simulink model "wrench_maats_simulator"  (R2025b)
settings: Solver=ode15s  StartTime=0.0  StopTime=100  FixedStep=1e-4  RelTol=1e-3
values from neighbouring files (symbols this model uses):
  Kd1 = 2    [parametrosCarga4x.m]
  x1_0 = xL0+q1_rot*[0;0;L1]    [parametrosCarga4x.m]
  x2_0 = xL0+q2_rot*[0;0;L2]    [parametrosCarga4x.m]
  x3_0 = xL0+q3_rot*[0;0;L3]    [parametrosCarga4x.m]
  x4_0 = xL0+q4_rot*[0;0;L4]    [parametrosCarga4x.m]
  xL0 = [0.8;0.8;0.1]    [parametrosCarga4x.m]
settings Model: Creator=ateveraz  LastModifiedBy=ateveraz

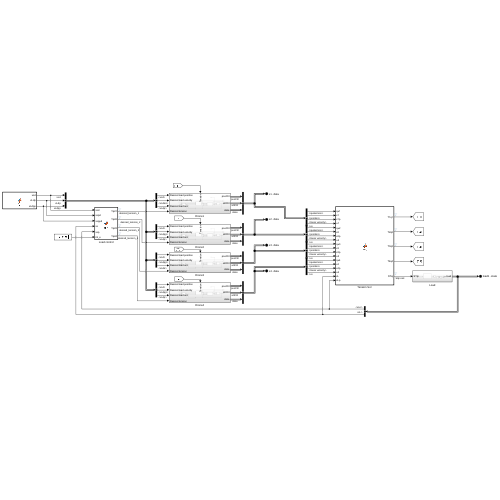
[thumbnail: Simulink's stored preview of the top-level diagram]
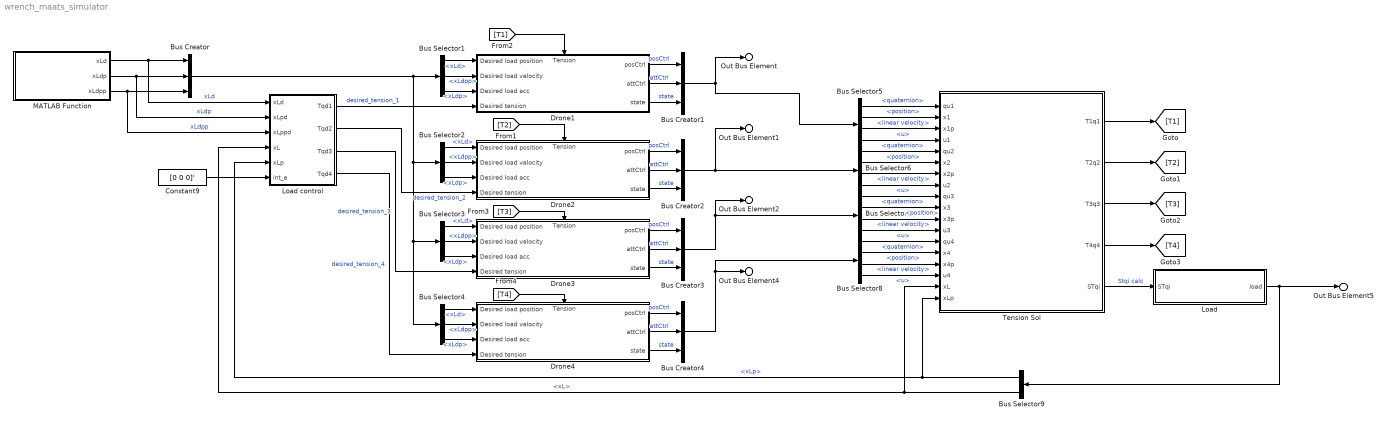
== system wrench_maats_simulator ==
  Bus Creator{,1..4} (5 alike) : BusCreator  Inputs=3
  Bus Selector{1..4} (4 alike) : BusSelector  OutputSignals=xLd,xLdpp,xLdp
  Bus Selector{5..8} (4 alike) : BusSelector  OutputSignals=state.quaternion,state.position,state.linear velocity,posCtrl.u
  Bus Selector9 : BusSelector  OutputSignals=xLp,xL
  Constant9 : Constant  Value=[0 0 0]'
  Drone1 : Subsystem
      settings: PortSchema="{\"entries\":[{\"content\":{\"sides\":[{\"content\":{\"connectorIds\":[\"In1\",\"In2\",\"In3\",\"In4\"]},\"type\":\"ConnectorPlacement.EquallySpacedRectSide\",\"uuid\":\"21103dfc-7bbe-40e0-9fc6-037905f1ea97\"},{\"content\":{\"connectorIds\":[\"Out1\",\"Out2\",\"Out3\"],\"side\":\"RIGHT\"},\"type\":\"ConnectorPlacement.EquallySpacedRectSide\",\"uuid\":\"5db0cf3b-93f2-491f-9cf6-07daf4674486\"},{\"content\":{\"connectorIds\":[\"In5\"],\"side\":\"TOP\"},\"type\":\"ConnectorPlacement.EquallySpacedRectSide\",\"uuid\":\"a4b55797-f354-4dcd-9bd0-022aba8efa3f\"}]},\"type\":\"ConnectorPlacement.EquallySpacedConnector\",\"uuid\":\"4e7ed67a-de76-4120-bfce-551a78690751\"}],\"packageUris\":[\"http://schema.mathworks.com/mf0/Connector/R2020b\"],\"version\":\"1.0\"}"
  Drone2 : Subsystem
      settings: PortSchema="{\"entries\":[{\"content\":{\"sides\":[{\"content\":{\"connectorIds\":[\"In1\",\"In2\",\"In3\",\"In4\"]},\"type\":\"ConnectorPlacement.EquallySpacedRectSide\",\"uuid\":\"21103dfc-7bbe-40e0-9fc6-037905f1ea97\"},{\"content\":{\"connectorIds\":[\"Out1\",\"Out2\",\"Out3\"],\"side\":\"RIGHT\"},\"type\":\"ConnectorPlacement.EquallySpacedRectSide\",\"uuid\":\"5db0cf3b-93f2-491f-9cf6-07daf4674486\"},{\"content\":{\"connectorIds\":[\"In5\"],\"side\":\"TOP\"},\"type\":\"ConnectorPlacement.EquallySpacedRectSide\",\"uuid\":\"a4b55797-f354-4dcd-9bd0-022aba8efa3f\"}]},\"type\":\"ConnectorPlacement.EquallySpacedConnector\",\"uuid\":\"4e7ed67a-de76-4120-bfce-551a78690751\"}],\"packageUris\":[\"http://schema.mathworks.com/mf0/Connector/R2020b\"],\"version\":\"1.0\"}"
  Drone3 : Subsystem
      settings: PortSchema="{\"entries\":[{\"content\":{\"sides\":[{\"content\":{\"connectorIds\":[\"In1\",\"In2\",\"In3\",\"In4\"]},\"type\":\"ConnectorPlacement.EquallySpacedRectSide\",\"uuid\":\"21103dfc-7bbe-40e0-9fc6-037905f1ea97\"},{\"content\":{\"connectorIds\":[\"Out1\",\"Out2\",\"Out3\"],\"side\":\"RIGHT\"},\"type\":\"ConnectorPlacement.EquallySpacedRectSide\",\"uuid\":\"5db0cf3b-93f2-491f-9cf6-07daf4674486\"},{\"content\":{\"connectorIds\":[\"In5\"],\"side\":\"TOP\"},\"type\":\"ConnectorPlacement.EquallySpacedRectSide\",\"uuid\":\"a4b55797-f354-4dcd-9bd0-022aba8efa3f\"}]},\"type\":\"ConnectorPlacement.EquallySpacedConnector\",\"uuid\":\"4e7ed67a-de76-4120-bfce-551a78690751\"}],\"packageUris\":[\"http://schema.mathworks.com/mf0/Connector/R2020b\"],\"version\":\"1.0\"}"
  Drone4 : Subsystem
      settings: PortSchema="{\"entries\":[{\"content\":{\"sides\":[{\"content\":{\"connectorIds\":[\"In1\",\"In2\",\"In3\",\"In4\"]},\"type\":\"ConnectorPlacement.EquallySpacedRectSide\",\"uuid\":\"21103dfc-7bbe-40e0-9fc6-037905f1ea97\"},{\"content\":{\"connectorIds\":[\"Out1\",\"Out2\",\"Out3\"],\"side\":\"RIGHT\"},\"type\":\"ConnectorPlacement.EquallySpacedRectSide\",\"uuid\":\"5db0cf3b-93f2-491f-9cf6-07daf4674486\"},{\"content\":{\"connectorIds\":[\"In5\"],\"side\":\"TOP\"},\"type\":\"ConnectorPlacement.EquallySpacedRectSide\",\"uuid\":\"a4b55797-f354-4dcd-9bd0-022aba8efa3f\"}]},\"type\":\"ConnectorPlacement.EquallySpacedConnector\",\"uuid\":\"4e7ed67a-de76-4120-bfce-551a78690751\"}],\"packageUris\":[\"http://schema.mathworks.com/mf0/Connector/R2020b\"],\"version\":\"1.0\"}"
  Load : Subsystem
  Load control : MATLAB Function  TreatAsAtomicUnit=on
  MATLAB Function : MATLAB Function  TreatAsAtomicUnit=on
  "Tension Sol " : MATLAB Function  TreatAsAtomicUnit=on
  Out Bus Element : Outport  PortName=x1  Element=data
  Out Bus Element1 : Outport  Port=2  PortName=x2  Element=data
  Out Bus Element2 : Outport  Port=3  PortName=x3  Element=data
  Out Bus Element4 : Outport  Port=4  PortName=x4  Element=data
  Out Bus Element5 : Outport  Port=5  PortName=load1  Element=state
  wires:
  Drone1/1(posCtrl) -> Bus Creator1/1  "posCtrl"
  Drone1/2(attCtrl) -> Bus Creator1/2  "attCtrl"
  Drone1/3(state) -> Bus Creator1/3  "state"
  MATLAB Function/1(xLd) -> Load control/1(xLd), Bus Creator/1  "xLd"
  MATLAB Function/2(xLdp) -> Load control/2(xLpd), Bus Creator/2  "xLdp"
  MATLAB Function/3(xLdpp) -> Load control/3(xLppd), Bus Creator/3  "xLdpp"
  Constant9/1 -> Load control/6(int_e)
  Load control/1(Tqd1) -> Drone1/4(Desired tension)  "desired_tension_1"
  Bus Selector1/1 -> Drone1/1(Desired load position)  "<xLd>"
  Bus Selector1/2 -> Drone1/2(Desired load velocity)  "<xLdpp>"
  Bus Selector1/3 -> Drone1/3(Desired load acc)  "<xLdp>"
  Bus Selector2/3 -> Drone2/3(Desired load acc)  "<xLdp>"
  Bus Selector2/2 -> Drone2/2(Desired load velocity)  "<xLdpp>"
  Bus Selector2/1 -> Drone2/1(Desired load position)  "<xLd>"
  Load control/2(Tqd2) -> Drone2/4(Desired tension)  "desired_tension_2"
  Load control/3(Tqd3) -> Drone3/4(Desired tension)  "desired_tension_3"
  Bus Creator/1 -> Bus Selector4/1, Bus Selector3/1, Bus Selector2/1, Bus Selector1/1
  Bus Selector3/2 -> Drone3/2(Desired load velocity)  "<xLdpp>"
  Bus Selector3/3 -> Drone3/3(Desired load acc)  "<xLdp>"
  Bus Selector3/1 -> Drone3/1(Desired load position)  "<xLd>"
  Bus Selector4/1 -> Drone4/1(Desired load position)  "<xLd>"
  Bus Selector4/3 -> Drone4/3(Desired load acc)  "<xLdp>"
  Bus Selector4/2 -> Drone4/2(Desired load velocity)  "<xLdpp>"
  Load control/4(Tqd4) -> Drone4/4(Desired tension)  "desired_tension_4"
  Bus Creator1/1 -> Bus Selector5/1, Out Bus Element/1
  Bus Creator2/1 -> Out Bus Element1/1, Bus Selector6/1
  Drone2/3(state) -> Bus Creator2/3  "state"
  Drone2/2(attCtrl) -> Bus Creator2/2  "attCtrl"
  Drone2/1(posCtrl) -> Bus Creator2/1  "posCtrl"
  Drone3/1(posCtrl) -> Bus Creator3/1  "posCtrl"
  Drone3/2(attCtrl) -> Bus Creator3/2  "attCtrl"
  Drone3/3(state) -> Bus Creator3/3  "state"
  Bus Creator3/1 -> Out Bus Element2/1, Bus Selector7/1
  Bus Creator4/1 -> Bus Selector8/1, Out Bus Element4/1
  Drone4/3(state) -> Bus Creator4/3  "state"
  Drone4/2(attCtrl) -> Bus Creator4/2  "attCtrl"
  Drone4/1(posCtrl) -> Bus Creator4/1  "posCtrl"
  [T2] -> Drone2/5(Tension)
  [T3] -> Drone3/5(Tension)
  [T4] -> Drone4/5(Tension)
  [T1] -> Drone1/5(Tension)
  "Tension Sol "/1(T1q1) -> [T1]
  "Tension Sol "/2(T2q2) -> [T2]
  Bus Selector9/2 -> "Tension Sol "/17(xL), Load control/4(xL)  "<xL>"
  "Tension Sol "/3(T3q3) -> [T3]
  Load/1(load) -> Out Bus Element5/1, Bus Selector9/1
  Bus Selector9/1 -> "Tension Sol "/18(xLp), Load control/5(xLp)  "<xLp>"
  "Tension Sol "/4(T4q4) -> [T4]
  "Tension Sol "/5(STqi) -> Load/1(STqi)  "Stqi calc"
  Bus Selector5/1 -> "Tension Sol "/1(qu1)  "<quaternion>"
  Bus Selector5/2 -> "Tension Sol "/2(x1)  "<position>"
  Bus Selector5/3 -> "Tension Sol "/3(x1p)  "<linear velocity>"
  Bus Selector5/4 -> "Tension Sol "/4(u1)  "<u>"
  Bus Selector6/1 -> "Tension Sol "/5(qu2)  "<quaternion>"
  Bus Selector6/2 -> "Tension Sol "/6(x2)  "<position>"
  Bus Selector6/3 -> "Tension Sol "/7(x2p)  "<linear velocity>"
  Bus Selector6/4 -> "Tension Sol "/8(u2)  "<u>"
  Bus Selector7/1 -> "Tension Sol "/9(qu3)  "<quaternion>"
  Bus Selector7/2 -> "Tension Sol "/10(x3)  "<position>"
  Bus Selector7/3 -> "Tension Sol "/11(x3p)  "<linear velocity>"
  Bus Selector7/4 -> "Tension Sol "/12(u3)  "<u>"
  Bus Selector8/1 -> "Tension Sol "/13(qu4)  "<quaternion>"
  Bus Selector8/2 -> "Tension Sol "/14(x4)  "<position>"
  Bus Selector8/3 -> "Tension Sol "/15(x4p)  "<linear velocity>"
  Bus Selector8/4 -> "Tension Sol "/16(u4)  "<u>"

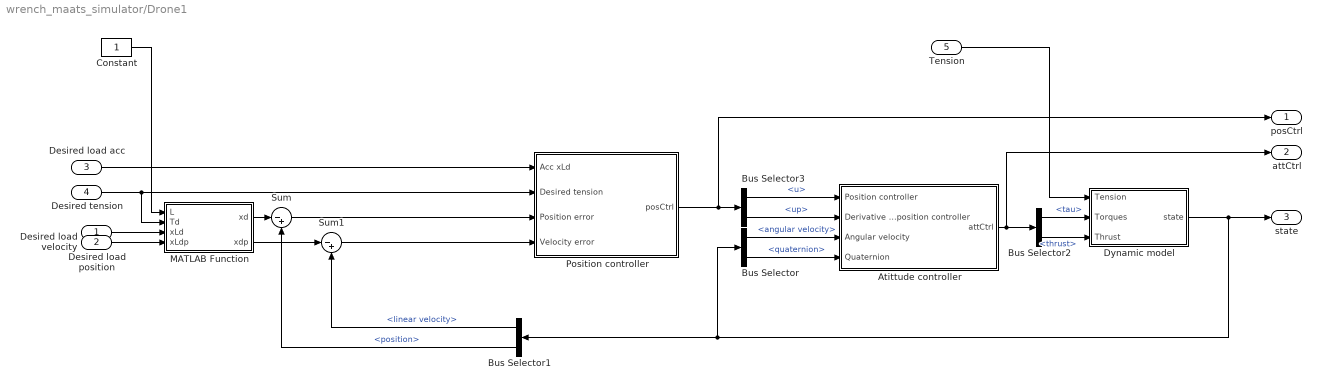
== system wrench_maats_simulator/Drone1 ==
  Desired load position : Inport
  Desired load velocity : Inport  Port=2
  Desired load acc : Inport  Port=3
  Desired tension : Inport  Port=4
  Tension : Inport  Port=5
  Atittude controller : Subsystem
  Bus Selector : BusSelector  OutputSignals=angular velocity,quaternion
  Bus Selector1 : BusSelector  OutputSignals=linear velocity,position
  Bus Selector2 : BusSelector  OutputSignals=tau,thrust
  Bus Selector3 : BusSelector  OutputSignals=u,up
  Constant : Constant
  Dynamic model : Subsystem
  MATLAB Function : MATLAB Function  TreatAsAtomicUnit=on
  Position controller : Subsystem
  Sum : Sum  Inputs=|-+
  Sum1 : Sum  Inputs=|-+
  posCtrl : Outport
  attCtrl : Outport  Port=2
  state : Outport  Port=3
  wires:
  Sum1/1 -> Position controller/4(Velocity error)
  Desired load velocity/1 -> MATLAB Function/4(xLdp)
  Bus Selector3/1 -> Atittude controller/1(Position controller)  "<u>"
  Bus Selector2/1 -> Dynamic model/2(Torques)  "<tau>"
  Atittude controller/1(attCtrl) -> attCtrl/1, Bus Selector2/1
  Desired tension/1 -> MATLAB Function/2(Td), Position controller/2(Desired tension)
  Desired load acc/1 -> Position controller/1(Acc xLd)
  Sum/1 -> Position controller/3(Position error)
  Bus Selector1/2 -> Sum/2  "<position>"
  Position controller/1(posCtrl) -> posCtrl/1, Bus Selector3/1
  Bus Selector2/2 -> Dynamic model/3(Thrust)  "<thrust>"
  Desired load position/1 -> MATLAB Function/3(xLd)
  Bus Selector1/1 -> Sum1/2  "<linear velocity>"
  Dynamic model/1(state) -> Bus Selector/1, Bus Selector1/1, state/1
  Bus Selector3/2 -> Atittude controller/2(Derivative position controller)  "<up>"
  MATLAB Function/1(xd) -> Sum/1
  MATLAB Function/2(xdp) -> Sum1/1
  Constant/1 -> MATLAB Function/1(L)
  Tension/1 -> Dynamic model/1(Tension)
  Bus Selector/1 -> Atittude controller/3(Angular velocity)  "<angular velocity>"
  Bus Selector/2 -> Atittude controller/4(Quaternion)  "<quaternion>"

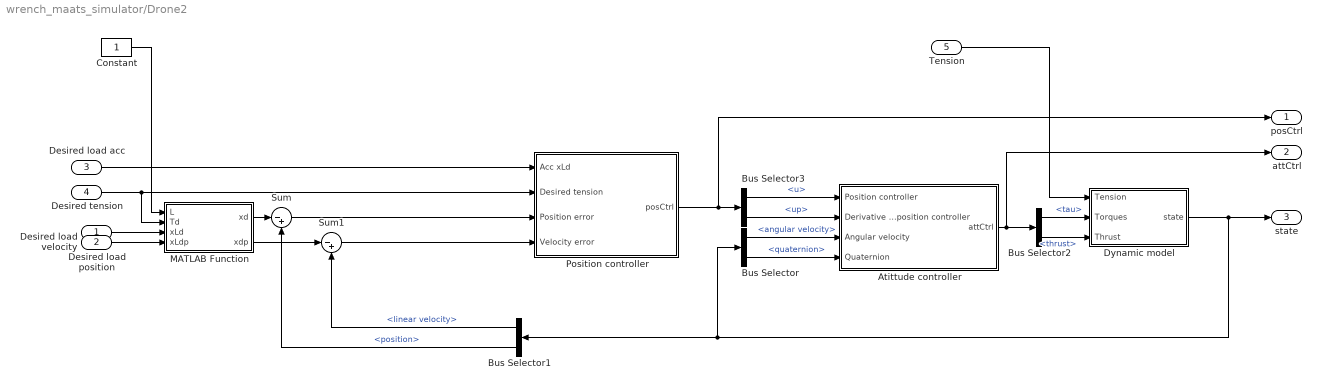
== system wrench_maats_simulator/Drone2 ==
  Desired load position : Inport
  Desired load velocity : Inport  Port=2
  Desired load acc : Inport  Port=3
  Desired tension : Inport  Port=4
  Tension : Inport  Port=5
  Atittude controller : Subsystem
  Bus Selector : BusSelector  OutputSignals=angular velocity,quaternion
  Bus Selector1 : BusSelector  OutputSignals=linear velocity,position
  Bus Selector2 : BusSelector  OutputSignals=tau,thrust
  Bus Selector3 : BusSelector  OutputSignals=u,up
  Constant : Constant
  Dynamic model : Subsystem
  MATLAB Function : MATLAB Function  TreatAsAtomicUnit=on
  Position controller : Subsystem
  Sum : Sum  Inputs=|-+
  Sum1 : Sum  Inputs=|-+
  posCtrl : Outport
  attCtrl : Outport  Port=2
  state : Outport  Port=3
  wires:
  Bus Selector/2 -> Atittude controller/4(Quaternion)  "<quaternion>"
  Bus Selector/1 -> Atittude controller/3(Angular velocity)  "<angular velocity>"
  Tension/1 -> Dynamic model/1(Tension)
  Constant/1 -> MATLAB Function/1(L)
  MATLAB Function/2(xdp) -> Sum1/1
  MATLAB Function/1(xd) -> Sum/1
  Bus Selector3/2 -> Atittude controller/2(Derivative position controller)  "<up>"
  Dynamic model/1(state) -> state/1, Bus Selector1/1, Bus Selector/1
  Bus Selector1/1 -> Sum1/2  "<linear velocity>"
  Desired load position/1 -> MATLAB Function/3(xLd)
  Bus Selector2/2 -> Dynamic model/3(Thrust)  "<thrust>"
  Position controller/1(posCtrl) -> Bus Selector3/1, posCtrl/1
  Bus Selector1/2 -> Sum/2  "<position>"
  Sum/1 -> Position controller/3(Position error)
  Desired load acc/1 -> Position controller/1(Acc xLd)
  Desired tension/1 -> Position controller/2(Desired tension), MATLAB Function/2(Td)
  Atittude controller/1(attCtrl) -> Bus Selector2/1, attCtrl/1
  Bus Selector2/1 -> Dynamic model/2(Torques)  "<tau>"
  Bus Selector3/1 -> Atittude controller/1(Position controller)  "<u>"
  Desired load velocity/1 -> MATLAB Function/4(xLdp)
  Sum1/1 -> Position controller/4(Velocity error)

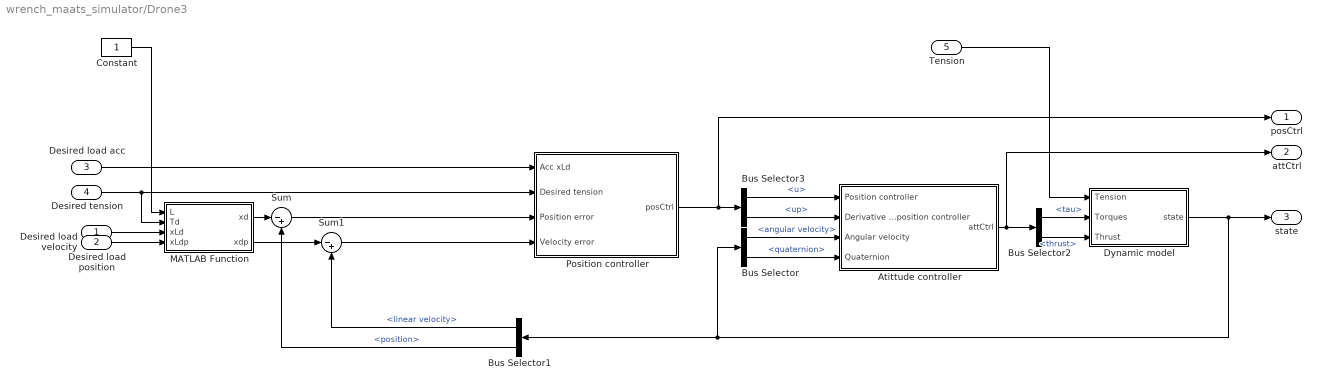
== system wrench_maats_simulator/Drone3 ==
  Desired load position : Inport
  Desired load velocity : Inport  Port=2
  Desired load acc : Inport  Port=3
  Desired tension : Inport  Port=4
  Tension : Inport  Port=5
  Atittude controller : Subsystem
  Bus Selector : BusSelector  OutputSignals=angular velocity,quaternion
  Bus Selector1 : BusSelector  OutputSignals=linear velocity,position
  Bus Selector2 : BusSelector  OutputSignals=tau,thrust
  Bus Selector3 : BusSelector  OutputSignals=u,up
  Constant : Constant
  Dynamic model : Subsystem
  MATLAB Function : MATLAB Function  TreatAsAtomicUnit=on
  Position controller : Subsystem
  Sum : Sum  Inputs=|-+
  Sum1 : Sum  Inputs=|-+
  posCtrl : Outport
  attCtrl : Outport  Port=2
  state : Outport  Port=3
  wires:
  Sum1/1 -> Position controller/4(Velocity error)
  Desired load velocity/1 -> MATLAB Function/4(xLdp)
  Bus Selector3/1 -> Atittude controller/1(Position controller)  "<u>"
  Bus Selector2/1 -> Dynamic model/2(Torques)  "<tau>"
  Atittude controller/1(attCtrl) -> attCtrl/1, Bus Selector2/1
  Desired tension/1 -> MATLAB Function/2(Td), Position controller/2(Desired tension)
  Desired load acc/1 -> Position controller/1(Acc xLd)
  Sum/1 -> Position controller/3(Position error)
  Bus Selector1/2 -> Sum/2  "<position>"
  Position controller/1(posCtrl) -> posCtrl/1, Bus Selector3/1
  Bus Selector2/2 -> Dynamic model/3(Thrust)  "<thrust>"
  Desired load position/1 -> MATLAB Function/3(xLd)
  Bus Selector1/1 -> Sum1/2  "<linear velocity>"
  Dynamic model/1(state) -> Bus Selector/1, Bus Selector1/1, state/1
  Bus Selector3/2 -> Atittude controller/2(Derivative position controller)  "<up>"
  MATLAB Function/1(xd) -> Sum/1
  MATLAB Function/2(xdp) -> Sum1/1
  Constant/1 -> MATLAB Function/1(L)
  Tension/1 -> Dynamic model/1(Tension)
  Bus Selector/1 -> Atittude controller/3(Angular velocity)  "<angular velocity>"
  Bus Selector/2 -> Atittude controller/4(Quaternion)  "<quaternion>"

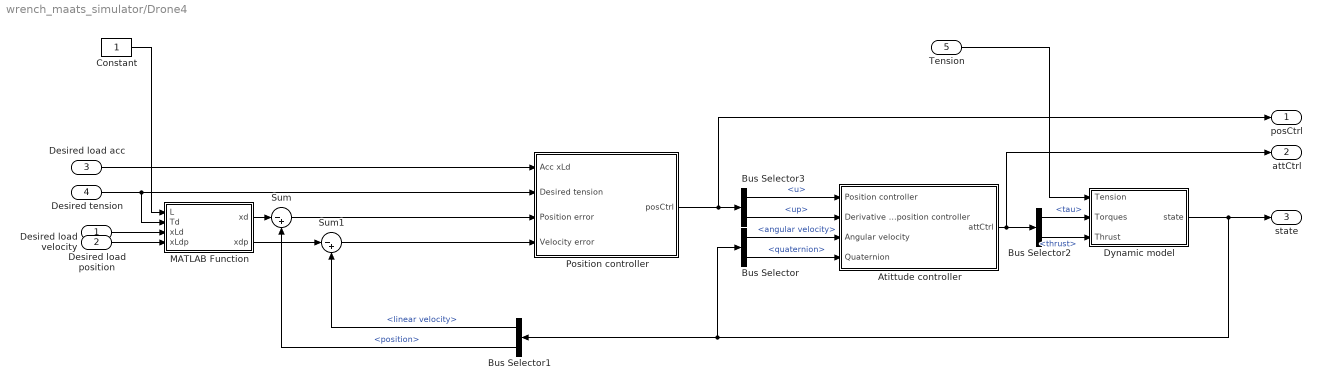
== system wrench_maats_simulator/Drone4 ==
  Desired load position : Inport
  Desired load velocity : Inport  Port=2
  Desired load acc : Inport  Port=3
  Desired tension : Inport  Port=4
  Tension : Inport  Port=5
  Atittude controller : Subsystem
  Bus Selector : BusSelector  OutputSignals=angular velocity,quaternion
  Bus Selector1 : BusSelector  OutputSignals=linear velocity,position
  Bus Selector2 : BusSelector  OutputSignals=tau,thrust
  Bus Selector3 : BusSelector  OutputSignals=u,up
  Constant : Constant
  Dynamic model : Subsystem
  MATLAB Function : MATLAB Function  TreatAsAtomicUnit=on
  Position controller : Subsystem
  Sum : Sum  Inputs=|-+
  Sum1 : Sum  Inputs=|-+
  posCtrl : Outport
  attCtrl : Outport  Port=2
  state : Outport  Port=3
  wires:
  Bus Selector/2 -> Atittude controller/4(Quaternion)  "<quaternion>"
  Bus Selector/1 -> Atittude controller/3(Angular velocity)  "<angular velocity>"
  Tension/1 -> Dynamic model/1(Tension)
  Constant/1 -> MATLAB Function/1(L)
  MATLAB Function/2(xdp) -> Sum1/1
  MATLAB Function/1(xd) -> Sum/1
  Bus Selector3/2 -> Atittude controller/2(Derivative position controller)  "<up>"
  Dynamic model/1(state) -> state/1, Bus Selector1/1, Bus Selector/1
  Bus Selector1/1 -> Sum1/2  "<linear velocity>"
  Desired load position/1 -> MATLAB Function/3(xLd)
  Bus Selector2/2 -> Dynamic model/3(Thrust)  "<thrust>"
  Position controller/1(posCtrl) -> Bus Selector3/1, posCtrl/1
  Bus Selector1/2 -> Sum/2  "<position>"
  Sum/1 -> Position controller/3(Position error)
  Desired load acc/1 -> Position controller/1(Acc xLd)
  Desired tension/1 -> Position controller/2(Desired tension), MATLAB Function/2(Td)
  Atittude controller/1(attCtrl) -> Bus Selector2/1, attCtrl/1
  Bus Selector2/1 -> Dynamic model/2(Torques)  "<tau>"
  Bus Selector3/1 -> Atittude controller/1(Position controller)  "<u>"
  Desired load velocity/1 -> MATLAB Function/4(xLdp)
  Sum1/1 -> Position controller/4(Velocity error)

== system wrench_maats_simulator/Load ==
  STqi : Inport
  Bus Creator : BusCreator  Inputs=2
  Constant : Constant  Value=xL0
  Embedded MATLAB Function3 : MATLAB Function  TreatAsAtomicUnit=on
  Integrator1 : Integrator  InitFcn=parametrosCarga4x  InitialCondition=[0;0;0]
  Integrator2 : Integrator  InitFcn=parametrosCarga4x  InitialConditionSource=external  InitialCondition=xL0
  load : Outport
  wires:
  Integrator2/1 -> Bus Creator/2  "xL"
  Embedded MATLAB Function3/1(xpp) -> Integrator1/1
  Constant/1 -> Integrator2/2
  STqi/1 -> Embedded MATLAB Function3/1(STq)
  Bus Creator/1 -> load/1
  Integrator1/1 -> Bus Creator/1, Integrator2/1  "xLp"

== system wrench_maats_simulator/Drone1/Atittude controller ==
  Position controller : Inport
  Derivative position controller : Inport  Port=2
  Angular velocity : Inport  Port=3
  Quaternion : Inport  Port=4
  Bus Creator : BusCreator  Inputs=3
  MATLAB System1 : MATLABSystem  System=AttitudeController  Kd=1  beta=0.3  gamma=10  rho=18  SimulateUsing=Code generation
      mask Type: AttitudeController
  MATLAB System2 : MATLABSystem  System=DesiredAttitude  SimulateUsing=Code generation
      mask Type: DesiredAttitude
  attCtrl : Outport
  wires:
  Angular velocity/1 -> MATLAB System2/3
  MATLAB System2/2 -> MATLAB System1/3
  Position controller/1 -> MATLAB System1/1, MATLAB System2/1
  Quaternion/1 -> MATLAB System2/4
  MATLAB System2/1 -> Bus Creator/3, MATLAB System1/2  "error quaternion"
  Derivative position controller/1 -> MATLAB System2/2
  MATLAB System1/2 -> Bus Creator/2  "thrust"
  Bus Creator/1 -> attCtrl/1
  MATLAB System1/1 -> Bus Creator/1  "tau"

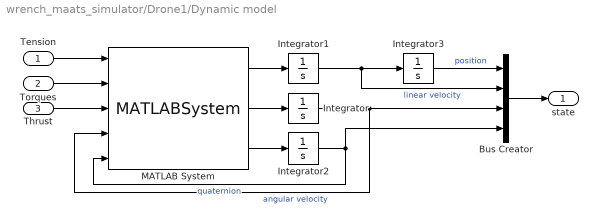
== system wrench_maats_simulator/Drone1/Dynamic model ==
  Tension : Inport
  Torques : Inport  Port=2
  Thrust : Inport  Port=3
  Bus Creator : BusCreator  Inputs=4
  Integrator : Integrator  InitialCondition=[0 0 0]'
  Integrator1 : Integrator  InitialCondition=[0 0 0]'
  Integrator2 : Integrator  InitialCondition=[1 0 0 0]'
  Integrator3 : Integrator  InitialCondition=x1_0
  MATLAB System : MATLABSystem  System=Modelx4  mass=mi  inertia_matrix=J  SimulateUsing=Code generation
      mask Type: Modelx4
  state : Outport
  wires:
  MATLAB System/1 -> Integrator1/1
  Integrator3/1 -> Bus Creator/1  "position"
  MATLAB System/3 -> Integrator2/1
  MATLAB System/2 -> Integrator/1
  Integrator2/1 -> MATLAB System/5, Bus Creator/4  "quaternion"
  Torques/1 -> MATLAB System/2
  Integrator1/1 -> Bus Creator/2, Integrator3/1  "linear velocity"
  Thrust/1 -> MATLAB System/3
  Integrator/1 -> MATLAB System/4, Bus Creator/3  "angular velocity"
  Bus Creator/1 -> state/1
  Tension/1 -> MATLAB System/1

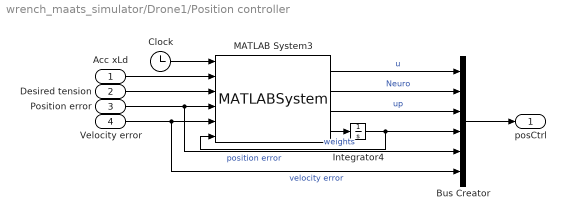
== system wrench_maats_simulator/Drone1/Position controller ==
  Acc xLd : Inport
  Desired tension : Inport  Port=2
  Position error : Inport  Port=3
  Velocity error : Inport  Port=4
  Bus Creator : BusCreator  Inputs=6
  Clock : Clock
  Integrator4 : Integrator  InitialCondition=zeros(3,15)
  MATLAB System3 : MATLABSystem  System=PositionController  Kd=Kd1  alpha=Alpha1  mass=mi  Gamma=Gamma1  kappa=2  k=10  N_neurons=15  center_range=1  eta_width=linspace(1,10,15)  SimulateUsing=Interpreted execution
      mask Type: PositionController
  posCtrl : Outport
  wires:
  Position error/1 -> MATLAB System3/4, Bus Creator/5  "position error"
  Integrator4/1 -> MATLAB System3/6, Bus Creator/4  "weights"
  Bus Creator/1 -> posCtrl/1
  Velocity error/1 -> MATLAB System3/5, Bus Creator/6  "velocity error"
  MATLAB System3/4 -> Integrator4/1
  MATLAB System3/1 -> Bus Creator/1  "u"
  MATLAB System3/2 -> Bus Creator/2  "Neuro"
  MATLAB System3/3 -> Bus Creator/3  "up"
  Clock/1 -> MATLAB System3/1
  Acc xLd/1 -> MATLAB System3/2
  Desired tension/1 -> MATLAB System3/3

== system wrench_maats_simulator/Drone2/Atittude controller ==
  Position controller : Inport
  Derivative position controller : Inport  Port=2
  Angular velocity : Inport  Port=3
  Quaternion : Inport  Port=4
  Bus Creator : BusCreator  Inputs=3
  MATLAB System1 : MATLABSystem  System=AttitudeController  Kd=1  beta=0.3  gamma=10  rho=18  SimulateUsing=Code generation
      mask Type: AttitudeController
  MATLAB System2 : MATLABSystem  System=DesiredAttitude  SimulateUsing=Code generation
      mask Type: DesiredAttitude
  attCtrl : Outport
  wires:
  MATLAB System1/1 -> Bus Creator/1  "tau"
  Bus Creator/1 -> attCtrl/1
  MATLAB System1/2 -> Bus Creator/2  "thrust"
  Derivative position controller/1 -> MATLAB System2/2
  MATLAB System2/1 -> MATLAB System1/2, Bus Creator/3  "error quaternion"
  Quaternion/1 -> MATLAB System2/4
  Position controller/1 -> MATLAB System2/1, MATLAB System1/1
  MATLAB System2/2 -> MATLAB System1/3
  Angular velocity/1 -> MATLAB System2/3

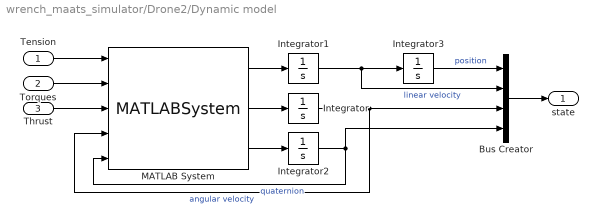
== system wrench_maats_simulator/Drone2/Dynamic model ==
  Tension : Inport
  Torques : Inport  Port=2
  Thrust : Inport  Port=3
  Bus Creator : BusCreator  Inputs=4
  Integrator : Integrator  InitialCondition=[0 0 0]'
  Integrator1 : Integrator  InitialCondition=[0 0 0]'
  Integrator2 : Integrator  InitialCondition=[1 0 0 0]'
  Integrator3 : Integrator  InitialCondition=x2_0
  MATLAB System : MATLABSystem  System=Modelx4  mass=mi  inertia_matrix=J  SimulateUsing=Code generation
      mask Type: Modelx4
  state : Outport
  wires:
  Tension/1 -> MATLAB System/1
  Bus Creator/1 -> state/1
  Integrator/1 -> Bus Creator/3, MATLAB System/4  "angular velocity"
  Thrust/1 -> MATLAB System/3
  Integrator1/1 -> Integrator3/1, Bus Creator/2  "linear velocity"
  Torques/1 -> MATLAB System/2
  Integrator2/1 -> Bus Creator/4, MATLAB System/5  "quaternion"
  MATLAB System/2 -> Integrator/1
  MATLAB System/3 -> Integrator2/1
  Integrator3/1 -> Bus Creator/1  "position"
  MATLAB System/1 -> Integrator1/1

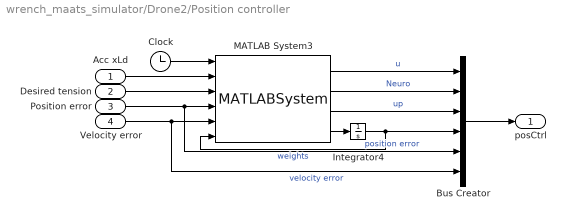
== system wrench_maats_simulator/Drone2/Position controller ==
  Acc xLd : Inport
  Desired tension : Inport  Port=2
  Position error : Inport  Port=3
  Velocity error : Inport  Port=4
  Bus Creator : BusCreator  Inputs=6
  Clock : Clock
  Integrator4 : Integrator  InitialCondition=zeros(3,15)
  MATLAB System3 : MATLABSystem  System=PositionController  Kd=Kd1  alpha=Alpha1  mass=mi  Gamma=Gamma1  kappa=2  k=10  N_neurons=15  center_range=1  eta_width=linspace(1,10,15)  SimulateUsing=Interpreted execution
      mask Type: PositionController
  posCtrl : Outport
  wires:
  Desired tension/1 -> MATLAB System3/3
  Acc xLd/1 -> MATLAB System3/2
  Clock/1 -> MATLAB System3/1
  MATLAB System3/3 -> Bus Creator/3  "up"
  MATLAB System3/2 -> Bus Creator/2  "Neuro"
  MATLAB System3/1 -> Bus Creator/1  "u"
  MATLAB System3/4 -> Integrator4/1
  Velocity error/1 -> Bus Creator/6, MATLAB System3/5  "velocity error"
  Bus Creator/1 -> posCtrl/1
  Integrator4/1 -> Bus Creator/4, MATLAB System3/6  "weights"
  Position error/1 -> Bus Creator/5, MATLAB System3/4  "position error"

== system wrench_maats_simulator/Drone3/Atittude controller ==
  Position controller : Inport
  Derivative position controller : Inport  Port=2
  Angular velocity : Inport  Port=3
  Quaternion : Inport  Port=4
  Bus Creator : BusCreator  Inputs=3
  MATLAB System1 : MATLABSystem  System=AttitudeController  Kd=1  beta=0.3  gamma=10  rho=18  SimulateUsing=Code generation
      mask Type: AttitudeController
  MATLAB System2 : MATLABSystem  System=DesiredAttitude  SimulateUsing=Code generation
      mask Type: DesiredAttitude
  attCtrl : Outport
  wires:
  Angular velocity/1 -> MATLAB System2/3
  MATLAB System2/2 -> MATLAB System1/3
  Position controller/1 -> MATLAB System1/1, MATLAB System2/1
  Quaternion/1 -> MATLAB System2/4
  MATLAB System2/1 -> Bus Creator/3, MATLAB System1/2  "error quaternion"
  Derivative position controller/1 -> MATLAB System2/2
  MATLAB System1/2 -> Bus Creator/2  "thrust"
  Bus Creator/1 -> attCtrl/1
  MATLAB System1/1 -> Bus Creator/1  "tau"

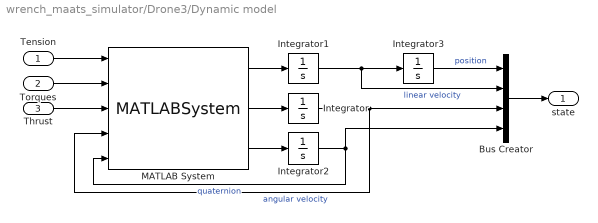
== system wrench_maats_simulator/Drone3/Dynamic model ==
  Tension : Inport
  Torques : Inport  Port=2
  Thrust : Inport  Port=3
  Bus Creator : BusCreator  Inputs=4
  Integrator : Integrator  InitialCondition=[0 0 0]'
  Integrator1 : Integrator  InitialCondition=[0 0 0]'
  Integrator2 : Integrator  InitialCondition=[1 0 0 0]'
  Integrator3 : Integrator  InitialCondition=x3_0
  MATLAB System : MATLABSystem  System=Modelx4  mass=mi  inertia_matrix=J  SimulateUsing=Code generation
      mask Type: Modelx4
  state : Outport
  wires:
  MATLAB System/1 -> Integrator1/1
  Integrator3/1 -> Bus Creator/1  "position"
  MATLAB System/3 -> Integrator2/1
  MATLAB System/2 -> Integrator/1
  Integrator2/1 -> MATLAB System/5, Bus Creator/4  "quaternion"
  Torques/1 -> MATLAB System/2
  Integrator1/1 -> Bus Creator/2, Integrator3/1  "linear velocity"
  Thrust/1 -> MATLAB System/3
  Integrator/1 -> MATLAB System/4, Bus Creator/3  "angular velocity"
  Bus Creator/1 -> state/1
  Tension/1 -> MATLAB System/1

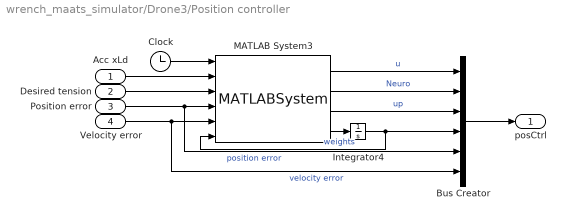
== system wrench_maats_simulator/Drone3/Position controller ==
  Acc xLd : Inport
  Desired tension : Inport  Port=2
  Position error : Inport  Port=3
  Velocity error : Inport  Port=4
  Bus Creator : BusCreator  Inputs=6
  Clock : Clock
  Integrator4 : Integrator  InitialCondition=zeros(3,15)
  MATLAB System3 : MATLABSystem  System=PositionController  Kd=Kd1  alpha=Alpha1  mass=mi  Gamma=Gamma1  kappa=2  k=10  N_neurons=15  center_range=1  eta_width=linspace(1,10,15)  SimulateUsing=Interpreted execution
      mask Type: PositionController
  posCtrl : Outport
  wires:
  Position error/1 -> MATLAB System3/4, Bus Creator/5  "position error"
  Integrator4/1 -> MATLAB System3/6, Bus Creator/4  "weights"
  Bus Creator/1 -> posCtrl/1
  Velocity error/1 -> MATLAB System3/5, Bus Creator/6  "velocity error"
  MATLAB System3/4 -> Integrator4/1
  MATLAB System3/1 -> Bus Creator/1  "u"
  MATLAB System3/2 -> Bus Creator/2  "Neuro"
  MATLAB System3/3 -> Bus Creator/3  "up"
  Clock/1 -> MATLAB System3/1
  Acc xLd/1 -> MATLAB System3/2
  Desired tension/1 -> MATLAB System3/3

== system wrench_maats_simulator/Drone4/Atittude controller ==
  Position controller : Inport
  Derivative position controller : Inport  Port=2
  Angular velocity : Inport  Port=3
  Quaternion : Inport  Port=4
  Bus Creator : BusCreator  Inputs=3
  MATLAB System1 : MATLABSystem  System=AttitudeController  Kd=1  beta=0.3  gamma=10  rho=18  SimulateUsing=Code generation
      mask Type: AttitudeController
  MATLAB System2 : MATLABSystem  System=DesiredAttitude  SimulateUsing=Code generation
      mask Type: DesiredAttitude
  attCtrl : Outport
  wires:
  MATLAB System1/1 -> Bus Creator/1  "tau"
  Bus Creator/1 -> attCtrl/1
  MATLAB System1/2 -> Bus Creator/2  "thrust"
  Derivative position controller/1 -> MATLAB System2/2
  MATLAB System2/1 -> MATLAB System1/2, Bus Creator/3  "error quaternion"
  Quaternion/1 -> MATLAB System2/4
  Position controller/1 -> MATLAB System2/1, MATLAB System1/1
  MATLAB System2/2 -> MATLAB System1/3
  Angular velocity/1 -> MATLAB System2/3

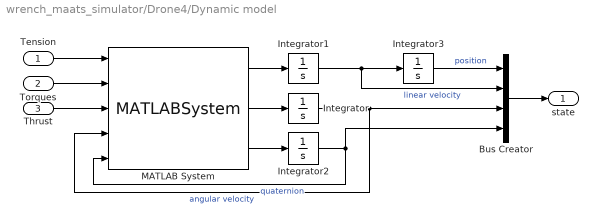
== system wrench_maats_simulator/Drone4/Dynamic model ==
  Tension : Inport
  Torques : Inport  Port=2
  Thrust : Inport  Port=3
  Bus Creator : BusCreator  Inputs=4
  Integrator : Integrator  InitialCondition=[0 0 0]'
  Integrator1 : Integrator  InitialCondition=[0 0 0]'
  Integrator2 : Integrator  InitialCondition=[1 0 0 0]'
  Integrator3 : Integrator  InitialCondition=x4_0
  MATLAB System : MATLABSystem  System=Modelx4  mass=mi  inertia_matrix=J  SimulateUsing=Code generation
      mask Type: Modelx4
  state : Outport
  wires:
  Tension/1 -> MATLAB System/1
  Bus Creator/1 -> state/1
  Integrator/1 -> Bus Creator/3, MATLAB System/4  "angular velocity"
  Thrust/1 -> MATLAB System/3
  Integrator1/1 -> Integrator3/1, Bus Creator/2  "linear velocity"
  Torques/1 -> MATLAB System/2
  Integrator2/1 -> Bus Creator/4, MATLAB System/5  "quaternion"
  MATLAB System/2 -> Integrator/1
  MATLAB System/3 -> Integrator2/1
  Integrator3/1 -> Bus Creator/1  "position"
  MATLAB System/1 -> Integrator1/1

== system wrench_maats_simulator/Drone4/Position controller ==
  Acc xLd : Inport
  Desired tension : Inport  Port=2
  Position error : Inport  Port=3
  Velocity error : Inport  Port=4
  Bus Creator : BusCreator  Inputs=6
  Clock : Clock
  Integrator4 : Integrator  InitialCondition=zeros(3,15)
  MATLAB System3 : MATLABSystem  System=PositionController  Kd=Kd1  alpha=Alpha1  mass=mi  Gamma=Gamma1  kappa=2  k=10  N_neurons=15  center_range=1  eta_width=linspace(1,10,15)  SimulateUsing=Interpreted execution
      mask Type: PositionController
  posCtrl : Outport
  wires:
  Desired tension/1 -> MATLAB System3/3
  Acc xLd/1 -> MATLAB System3/2
  Clock/1 -> MATLAB System3/1
  MATLAB System3/3 -> Bus Creator/3  "up"
  MATLAB System3/2 -> Bus Creator/2  "Neuro"
  MATLAB System3/1 -> Bus Creator/1  "u"
  MATLAB System3/4 -> Integrator4/1
  Velocity error/1 -> Bus Creator/6, MATLAB System3/5  "velocity error"
  Bus Creator/1 -> posCtrl/1
  Integrator4/1 -> Bus Creator/4, MATLAB System3/6  "weights"
  Position error/1 -> Bus Creator/5, MATLAB System3/4  "position error"

== matlab function wrench_maats_simulator/Drone4/MATLAB Function ==
  data: L input; xd output; Td input; xLd input; xLdp input; xdp output
function [xd, xdp] = fcn(L,  Td, xLd, xLdp)
    alpha = zeros(3,1);
    if (norm(Td)~=0)
        alpha = Td/norm(Td);
    end
    xd = xLd - L*alpha;
    xdp = xLdp;
end

== matlab function wrench_maats_simulator/Load/Embedded MATLAB Function3 ==
  settings: updateMethod=CONTINUOUS  sampleTime=0.025
  data: STq input; xpp output
function xpp = DinamicaPos(STq)
%% Datos Dinámica
 mL = 0.225;
ez = [0;0;1];
g = 9.81*ez;

%% Dinámica
xpp = STq/mL + g;

end

== matlab function wrench_maats_simulator/Tension Sol  ==
  data: qu1 input; x1 input size=3; x1p input size=3; u1 input; qu2 input; x2 input size=3; x2p input size=3; u2 input; qu3 input; x3 input size=3; x3p input size=3; u3 input; qu4 input; x4 input; x4p input; u4 input; xL input size=3; xLp input size=3; T1q1 output size=3; T2q2 output size=3; T3q3 output size=3; T4q4 output; STqi output size=3
function [T1q1,T2q2,T3q3,T4q4,STqi] = fcn(qu1,x1,x1p,u1,qu2,x2,x2p,u2,qu3,x3,x3p,u3,qu4,x4,x4p,u4,xL,xLp)
%function [T1q1,T2q2,T3q3,T4q4,STqi] = fcn(qu1,qu2,qu3,qu4,xL,xLp,x1,x1p,u1,x2,x2p,u2,x3,x3p,u3,x4,x4p,u4)

L1=1;
L2=1;
L3=1;
L4=1;
mi=0.4;
mL=0.225;
e3=[0;0;1];

%% Calcular las qis

d1 = (xL-x1)/L1; %qi's
d2 = (xL-x2)/L2; 
d3 = (xL-x3)/L3;
d4 = (xL-x4)/L4;


n1 = norm(d1); 
n2 = norm(d2); 
n3 = norm(d3);
n4 = norm(d4);

q1 = d1/n1; %qi's
q2 = d2/n2;
q3 = d3/n3;
q4 = d4/n4;

d1p = (xLp-x1p)/(L1);
d2p = (xLp-x2p)/(L2);
d3p = (xLp-x3p)/(L3);
d4p = (xLp-x4p)/(L4);

% d1p = (xLp-x1p)/(L1*n1)+d1*(d1'*dp1)/(L1*n1);
% d2p = (xLp-x2p)/(L2*n2);
% d3p = (xLp-x3p)/(L3*n3);
% d4p = (xLp-x4p)/(L4*n4);
% 
q1p = d1p/n1-d1*(d1'*d1p)/(n1^3); %%% estas eran las que usaba Fatima
q2p = d2p/n2-d2*(d2'*d2p)/(n2^3);
q3p = d3p/n3-d3*(d3'*d3p)/(n3^3);
q4p = d4p/n4-d4*(d4'*d4p)/(n4^3);

% q1p=d1p;
% q2p=d2p;
% q3p=d3p;
% q4p=d4p;

% q1pp = d1pp/n1-d1*(d1'*d1p)/(n1^3);
% q2pp = d2pp/n2-d2*(d2'*d2p)/(n2^3);
% q3pp = d3pp/n3-d3*(d3'*d3p)/(n3^3);
% q4pp = d4pp/n4-d4*(d4'*d4p)/(n4^3);

%% Calcular las Tis %%%%%%%% aqui voy para 4
md = (mL/mi)+1;

M = (1/mL)*[md,     q1'*q2, q1'*q3,  q1'*q4;
            q2'*q1, md,     q2'*q3,  q2'*q4;
            q3'*q1, q3'*q2, md,      q3'*q4;
            q4'*q1, q4'*q2, q4'*q3,  md];

eig(M);
% (nd1')*q1p

% ddds =[(-1/mi)*(q1')*u1+L1*(q1p')*q1p;
%        (-1/mi)*(q2')*u2+L2*(q2p')*q2p;
%        (-1/mi)*(q3')*u3+L3*(q3p')*q3p];

ddds =[(-1/mi)*(q1')*norm(u1)*qToR(qu1)*e3+L1*(q1p')*q1p;
       (-1/mi)*(q2')*norm(u2)*qToR(qu2)*e3+L2*(q2p')*q2p;
       (-1/mi)*(q3')*norm(u3)*qToR(qu3)*e3+L3*(q3p')*q3p;
       (-1/mi)*(q4')*norm(u4)*qToR(qu4)*e3+L4*(q4p')*q4p];

% T = zeros(3,1);
T = pinv(M)*ddds;

if T(1)<=0
    t1=T(1)
    T(1)=0;
end

if T(2)<=0
    t2=T(2)
    T(2)=0;
end

if T(3)<=0
    t3=T(3)
    T(3)=0;
end

if T(4)<=0
    t4=T(4)
    T(4)=0;
end


%% Fuerza en carga
T1q1=T(1)*q1;
T2q2=T(2)*q2;
T3q3=T(3)*q3;
T4q4=T(4)*q4;


STqi = T(1)*q1+T(2)*q2+T(3)*q3+T(4)*q4;
% fdL = zeros(3,1);
end

== matlab function wrench_maats_simulator/Load control ==
  data: xLd input; xLpd input; xLppd input; xL input; xLp input; Tqd1 output; Tqd2 output; Tqd3 output; int_e input; Tqd4 output
function [Tqd1,Tqd2,Tqd3,Tqd4] = fcn(xLd,xLpd,xLppd,xL,xLp,int_e)
    mL = 0.225;
    g  = [0;0;9.81];

    kpl = 1*diag([1,1,1]);
    kdl = 0.5*diag([1,1,1]);
    kil = 0*diag([1,1,1]);

    % Control de carga
    uL = - mL * (g + xLppd) - kpl * (xL - xLd)  - kdl * (xLp - xLpd) - kil * int_e;

    % Tension allocation
    Tqd2 = -(mL/4) * rotz(65)  * roty(-35) * g;
    Tqd3 = -(mL/4) * rotz(155) * roty(-35) * g;
    Tqd4 = -(mL/4) * rotz(245) * roty(-35) * g;

    Tqd1 = - uL + (Tqd2 + Tqd3 + Tqd4);
end

== matlab function wrench_maats_simulator/MATLAB Function ==
  data: xLd output; xLdp output; xLdpp output
function [xLd, xLdp, xLdpp] = fcn()
    xLd = [1 1 0]';
    xLdp = zeros(3,1);
    xLdpp = zeros(3,1);
end

== matlab function wrench_maats_simulator/Drone1/MATLAB Function ==
  data: L input; xd output; Td input; xLd input; xLdp input; xdp output
function [xd, xdp] = fcn(L,  Td, xLd, xLdp)
    alpha = zeros(3,1);
    if (norm(Td)~=0)
        alpha = Td/norm(Td);
    end
    xd = xLd - L*alpha;
    xdp = xLdp;
end

== matlab function wrench_maats_simulator/Drone2/MATLAB Function ==
  data: L input; xd output; Td input; xLd input; xLdp input; xdp output
function [xd, xdp] = fcn(L,  Td, xLd, xLdp)
    alpha = zeros(3,1);
    if (norm(Td)~=0)
        alpha = Td/norm(Td);
    end
    xd = xLd - L*alpha;
    xdp = xLdp;
end

== matlab function wrench_maats_simulator/Drone3/MATLAB Function ==
  data: L input; xd output; Td input; xLd input; xLdp input; xdp output
function [xd, xdp] = fcn(L,  Td, xLd, xLdp)
    alpha = zeros(3,1);
    if (norm(Td)~=0)
        alpha = Td/norm(Td);
    end
    xd = xLd - L*alpha;
    xdp = xLdp;
end
